simulink model "NSDselect_NoHeater_fractional"  (R2017b)
settings: Solver=ode4  StartTime=0.0  StopTime=720  FixedStep=1  RelTol=1e-3  EnableMultiTasking=on
libraries: dspsrcs4 x1
settings Model: Creator=dt  LastModifiedBy=dell
settings DataIOCC: LimitDataPoints=on
settings OptimizationCC: LifeSpan=inf
settings DebuggingCC: AllowSymbolicDim=off  SFUnexpectedBacktrackingDiag=warning  SFNoUnconditionalDefaultTransitionDiag=warning  SFExecutionAtInitializationDiag=none
settings ModelReferenceCC: PropagateSignalLabelsOutOfModel=off
settings CodeAppCC: StateflowObjectComments=on
settings GRTTargetCC: TargetLangStandard=C89/C90 (ANSI)
settings ConfigComp: CovMetricSettings=dw  CovHtmlReporting=on  CovSaveCumulativeToWorkspaceVar=on  CovSaveSingleToWorkspaceVar=on  CovExternalEMLEnable=off

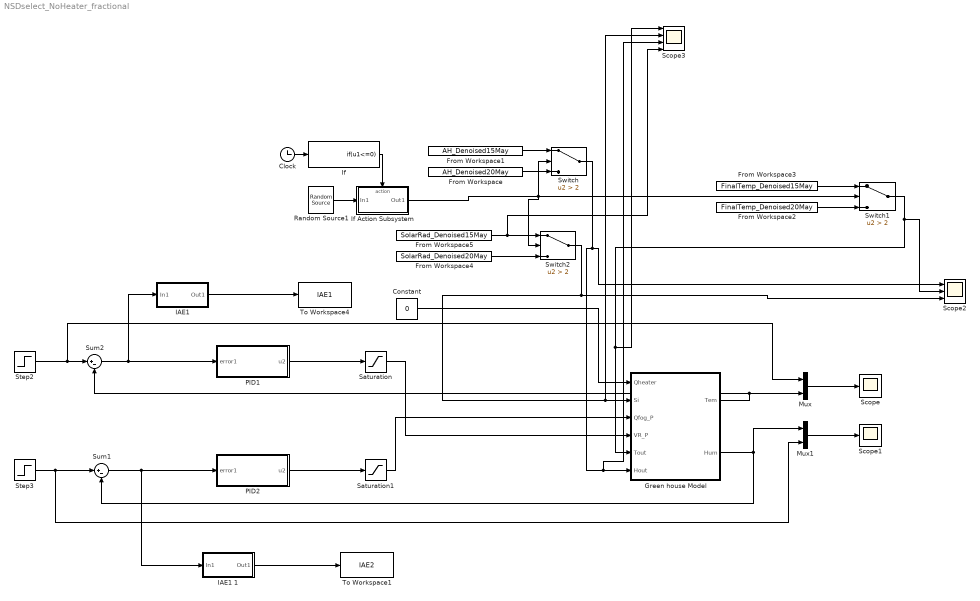
== system NSDselect_NoHeater_fractional ==
  Clock : Clock
  Constant : Constant  Value=0
  From Workspace : FromWorkspace  VariableName=AH_Denoised20May  SampleTime=0
  From Workspace1 : FromWorkspace  VariableName=AH_Denoised15May  SampleTime=0
  From Workspace2 : FromWorkspace  VariableName=FinalTemp_Denoised20May  SampleTime=0
  From Workspace3 : FromWorkspace  VariableName=FinalTemp_Denoised15May  SampleTime=0
  From Workspace4 : FromWorkspace  VariableName=SolarRad_Denoised20May  SampleTime=0
  From Workspace5 : FromWorkspace  VariableName=SolarRad_Denoised15May  SampleTime=0
  Green house Model : Subsystem
  "IAE1 " : Subsystem
      mask help:
      | IAE performacne index
      |
      | output = int |input| dt
      mask Display:
      | disp('IAE')
      | port_label('input',1,'e')
      | port_label('output',1,'iae')
  IAE1 1 : Subsystem
      mask help:
      | IAE performacne index
      |
      | output = int |input| dt
      mask Display:
      | disp('IAE')
      | port_label('input',1,'e')
      | port_label('output',1,'iae')
  If : If  IfExpression=u1<=0  ShowElse=off
  If Action Subsystem : Subsystem  TreatAsAtomicUnit=on
  Mux : Mux  Inputs=2
  Mux1 : Mux  Inputs=2
  PID1 : Subsystem
  PID2 : Subsystem
  Random Source1 : dspsrcs4/Random Source  SrcType=Uniform  NormMethod=Ziggurat  CltLength=12  MinVal=0  MaxVal=4  MeanVal=0  VarVal=1  RepMode=Not repeatable  rawSeed=1  IsInherit=off  SampMode=Discrete  SampTime=1  SampFrame=1  DataType=Double  OutComplex=Real  OutputFrames=off
  Saturation : Saturate  UpperLimit=1  LowerLimit=0
  Saturation1 : Saturate  UpperLimit=1  LowerLimit=0
  Scope : Scope
  Scope1 : Scope
  Scope2 : Scope  NumInputPorts=3
  Scope3 : Scope  NumInputPorts=4
  Step2 : Step  Time=0  After=28  SampleTime=0
  Step3 : Step  Time=0  After=24  SampleTime=0
  Sum1 : Sum  Inputs=|+-
  Sum2 : Sum  Inputs=|+-
  Switch : Switch  Criteria=u2 > Threshold  Threshold=2
  Switch1 : Switch  Criteria=u2 > Threshold  Threshold=2
  Switch2 : Switch  Criteria=u2 > Threshold  Threshold=2
  To Workspace1 : ToWorkspace  VariableName=IAE2  SampleTime=-1
      settings: Save2DSignal=2-D array (concatenate along first dimension)
  To Workspace4 : ToWorkspace  VariableName=IAE1  SampleTime=-1
      settings: Save2DSignal=2-D array (concatenate along first dimension)
  wires:
  Saturation/1 -> Green house Model/4(VR_P)
  Saturation1/1 -> Green house Model/3(Qfog_P)
  Constant/1 -> Green house Model/1(Qheater)
  Switch/1 -> Scope2/1, Scope3/3, Green house Model/6(Hout)
  Switch1/1 -> Scope2/2, Scope3/1, Green house Model/5(Tout)
  Switch2/1 -> Scope2/3, Scope3/2, Green house Model/2(Si)
  Green house Model/2(Hum) -> Mux1/1, Sum1/2
  Green house Model/1(Tem) -> Mux/2, Sum2/2
  Step2/1 -> Mux/1, Sum2/1
  Mux/1 -> Scope/1
  Mux1/1 -> Scope1/1
  Step3/1 -> Mux1/2, Sum1/1
  "IAE1 "/1(Out1) -> To Workspace4/1
  IAE1 1/1(Out1) -> To Workspace1/1
  PID1/1(u2) -> Saturation/1
  PID2/1(u2) -> Saturation1/1
  Sum2/1 -> PID1/1(error1), "IAE1 "/1(In1)
  Sum1/1 -> PID2/1(error1), IAE1 1/1(In1)
  If Action Subsystem/1(Out1) -> Switch2/2, Switch1/2, Switch/2
  From Workspace/1 -> Switch/3
  From Workspace1/1 -> Switch/1
  From Workspace2/1 -> Switch1/3
  From Workspace3/1 -> Switch1/1
  From Workspace4/1 -> Switch2/3
  From Workspace5/1 -> Scope3/4, Switch2/1
  Random Source1/1 -> If Action Subsystem/1(In1)
  If/1 -> If Action Subsystem/Action
  Clock/1 -> If/1

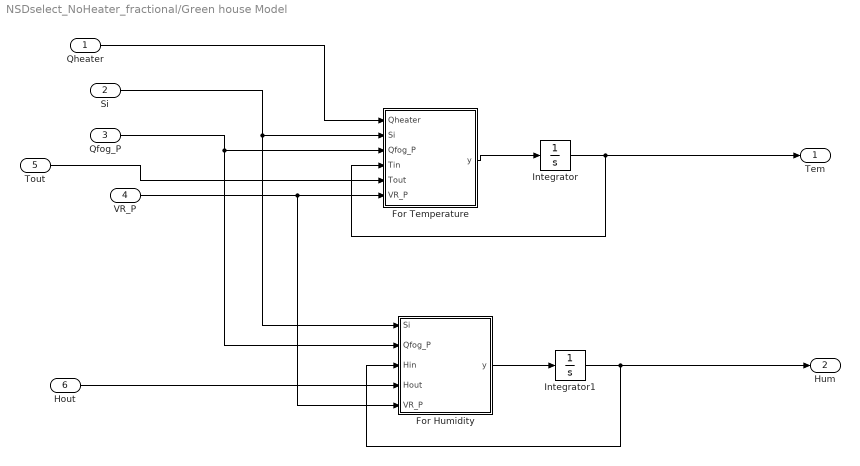
== system NSDselect_NoHeater_fractional/Green house Model ==
  Qheater : Inport
  Si : Inport  Port=2
  Qfog_P : Inport  Port=3
  VR_P : Inport  Port=4
  Tout : Inport  Port=5
  Hout : Inport  Port=6
  For Humidity : MATLAB Function  TreatAsAtomicUnit=on
  For Temperature : MATLAB Function  TreatAsAtomicUnit=on
  Integrator : Integrator  InitialCondition=30
  Integrator1 : Integrator  InitialCondition=18
  Tem : Outport
  Hum : Outport  Port=2
  wires:
  For Temperature/1(y) -> Integrator/1
  Integrator/1 -> Tem/1, For Temperature/4(Tin)
  VR_P/1 -> For Humidity/5(VR_P), For Temperature/6(VR_P)
  Si/1 -> For Humidity/1(Si), For Temperature/2(Si)
  Integrator1/1 -> Hum/1, For Humidity/3(Hin)
  For Humidity/1(y) -> Integrator1/1
  Qfog_P/1 -> For Humidity/2(Qfog_P), For Temperature/3(Qfog_P)
  Qheater/1 -> For Temperature/1(Qheater)
  Tout/1 -> For Temperature/5(Tout)
  Hout/1 -> For Humidity/4(Hout)

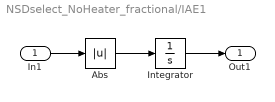
== system NSDselect_NoHeater_fractional/IAE1  ==
  In1 : Inport
  Abs : Abs
  Integrator : Integrator
  Out1 : Outport
  wires:
  In1/1 -> Abs/1
  Integrator/1 -> Out1/1
  Abs/1 -> Integrator/1

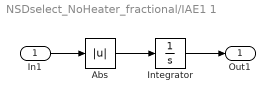
== system NSDselect_NoHeater_fractional/IAE1 1 ==
  In1 : Inport
  Abs : Abs
  Integrator : Integrator
  Out1 : Outport
  wires:
  In1/1 -> Abs/1
  Integrator/1 -> Out1/1
  Abs/1 -> Integrator/1

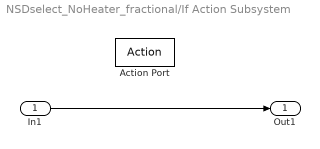
== system NSDselect_NoHeater_fractional/If Action Subsystem ==
  In1 : Inport
  Action Port : ActionPort  ActionType=then
  Out1 : Outport
  wires:
  In1/1 -> Out1/1

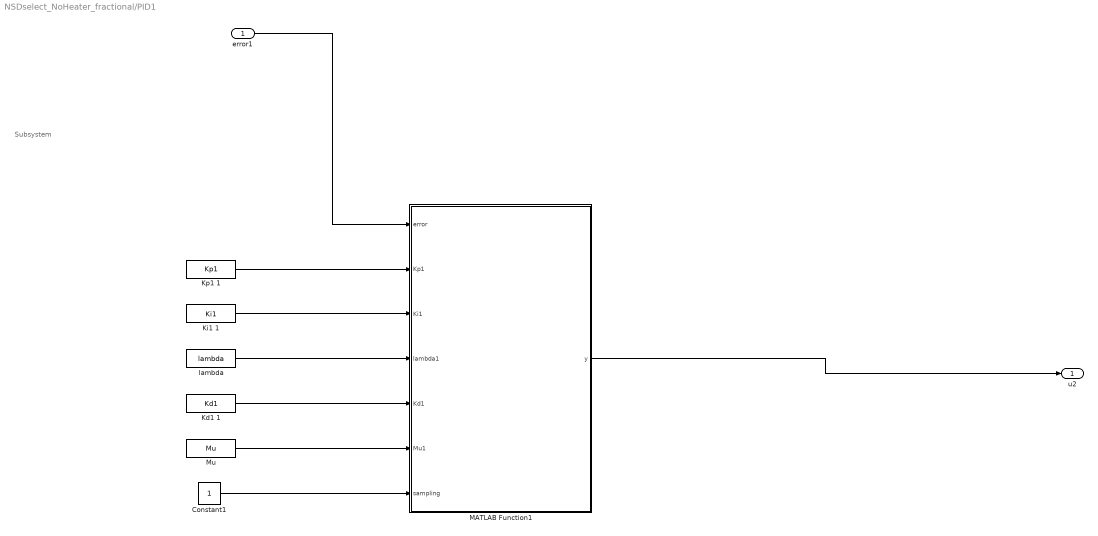
== system NSDselect_NoHeater_fractional/PID1 ==
  note: Subsystem
  error1 : Inport
  Constant1 : Constant
  Kd1 1 : FromWorkspace  VariableName=Kd1  OutDataTypeStr=double  SampleTime=0
  Ki1 1 : FromWorkspace  VariableName=Ki1  OutDataTypeStr=double  SampleTime=0
  Kp1 1 : FromWorkspace  VariableName=Kp1  OutDataTypeStr=double  SampleTime=0
  MATLAB Function1 : MATLAB Function  TreatAsAtomicUnit=on
  "Mu " : FromWorkspace  VariableName=Mu  OutDataTypeStr=double  SampleTime=0
  "lambda " : FromWorkspace  VariableName=lambda  OutDataTypeStr=double  SampleTime=0
  u2 : Outport
  wires:
  MATLAB Function1/1(y) -> u2/1
  "Mu "/1 -> MATLAB Function1/6(Mu1)
  "lambda "/1 -> MATLAB Function1/4(lambda1)
  Constant1/1 -> MATLAB Function1/7(sampling)
  Ki1 1/1 -> MATLAB Function1/3(Ki1)
  Kd1 1/1 -> MATLAB Function1/5(Kd1)
  Kp1 1/1 -> MATLAB Function1/2(Kp1)
  error1/1 -> MATLAB Function1/1(error)

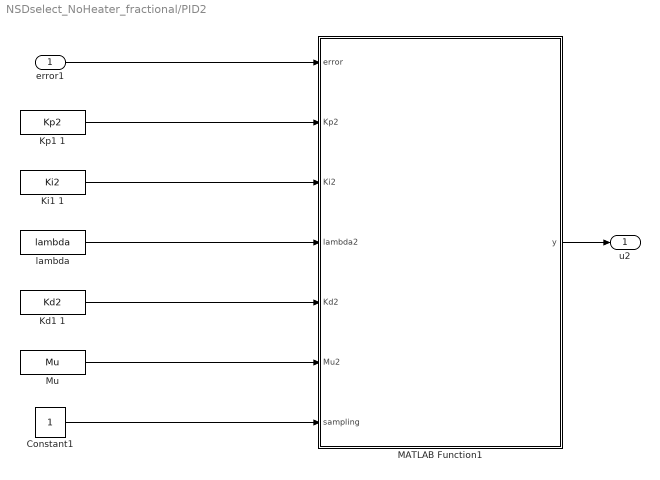
== system NSDselect_NoHeater_fractional/PID2 ==
  error1 : Inport
  Constant1 : Constant
  Kd1 1 : FromWorkspace  VariableName=Kd2  OutDataTypeStr=double  SampleTime=0
  Ki1 1 : FromWorkspace  VariableName=Ki2  OutDataTypeStr=double  SampleTime=0
  Kp1 1 : FromWorkspace  VariableName=Kp2  OutDataTypeStr=double  SampleTime=0
  MATLAB Function1 : MATLAB Function  TreatAsAtomicUnit=on
  "Mu " : FromWorkspace  VariableName=Mu  OutDataTypeStr=double  SampleTime=0
  "lambda " : FromWorkspace  VariableName=lambda  OutDataTypeStr=double  SampleTime=0
  u2 : Outport
  wires:
  Kp1 1/1 -> MATLAB Function1/2(Kp2)
  Ki1 1/1 -> MATLAB Function1/3(Ki2)
  Kd1 1/1 -> MATLAB Function1/5(Kd2)
  "lambda "/1 -> MATLAB Function1/4(lambda2)
  "Mu "/1 -> MATLAB Function1/6(Mu2)
  MATLAB Function1/1(y) -> u2/1
  Constant1/1 -> MATLAB Function1/7(sampling)
  error1/1 -> MATLAB Function1/1(error)

== matlab function NSDselect_NoHeater_fractional/Green house Model/For Humidity ==
  data: Si input; Qfog_P input; Hin input; Hout input; VR_P input; y output
function y = fcn(Si,Qfog_P,Hin,Hout,VR_P)
C0=-324.67;
UA=29.8;
tv=3.41;
V_V=13.3;
alpha_dash=0.0033;

y=V_V*Qfog_P+(alpha_dash*Si)-(VR_P/tv)*(Hin-Hout);

== matlab function NSDselect_NoHeater_fractional/Green house Model/For Temperature ==
  data: Qheater input; y output; Si input; Qfog_P input; Tin input; Tout input; VR_P input
function y = fcn(Qheater,Si,Qfog_P,Tin,Tout,VR_P)
C0=-324.67;
UA=29.8;
tv=3.41;
lambda_dash=465;
y=(1/C0)*(Qheater+Si-(lambda_dash*Qfog_P))-((VR_P/tv)+(UA/C0))*(Tin-Tout);

== matlab function NSDselect_NoHeater_fractional/PID2/MATLAB Function1 ==
  data: error input; y output; Kp2 input; Ki2 input; lambda2 input; Kd2 input; Mu2 input; sampling input
function y = fcn(error,Kp2,Ki2,lambda2,Kd2,Mu2,sampling)
%#codegen
lambda2 = lambda2*(-1);
diff = fgl_deriv(Mu2,error,sampling);
integrate = fgl_deriv(lambda2,error,sampling);
y = (Kp2*error + Kd2*diff + Ki2*(integrate));
end

function Y = fgl_deriv( a, y, h )
    n  = numel(y);
    J  = 0:(n-1);
    G1 = gamma( J+1 );
    G2 = gamma( a+1-J );
    s  = (-1) .^ J;
    M  = tril( ones(n) );
    R  = toeplitz( y(:)' );
    T  = meshgrid( (gamma(a+1)/(h^a)) * s ./ (G1.*G2) );
    Y  = reshape(sum(R.*M.*T,2), size(y));
end

== matlab function NSDselect_NoHeater_fractional/PID1/MATLAB Function1 ==
  data: error input; y output; Kp1 input; Ki1 input; lambda1 input; Kd1 input; Mu1 input; sampling input
function y = fcn(error,Kp1,Ki1,lambda1,Kd1,Mu1,sampling)
%#codegen
lambda1 = lambda1.*(-1);
diff = fgl_deriv(Mu1,error,sampling);
integrate = fgl_deriv(lambda1,error,sampling);
y = (Kp1.*error + Kd1.*diff+Ki1*integrate );
end

function Y = fgl_deriv( a, y, h )
    n  = numel(y);
    J  = 0:(n-1);
    G1 = gamma( J+1 );
    G2 = gamma( a+1-J );
    s  = (-1) .^ J;
    M  = tril( ones(n) );
    R  = toeplitz( y(:)' );
    T  = meshgrid( (gamma(a+1)/(h^a)) * s ./ (G1.*G2) );
    Y  = reshape(sum(R.*M.*T,2), size(y));
end
